simulink model "Arti_DeltaSM_Control_Fricc"  (R2014a)
settings: Solver=ode15s  StartTime=0.0  StopTime=6  FixedStep=0.0005  RelTol=1e-3
PreLoadFcn:
  | Fs=0.001;
  | Fc=0.0005;
undefined symbols (not defined in the file or in its folder): X, Y, Z
libraries: sm_lib x238, Fricciones x15, nesl_utility x10, simulink x3
(part 6 of 6)

== system Arti_DeltaSM_Control_Fricc/DeltaSM/BaseMovil/acopleBaseMovilAntebrazo_3_RIGID/ball_Uniball_1_RIGID ==
  ReferenceFrame : sm_lib/Frames and Transforms/Reference Frame  BlockFunction=simmechanics.library.frames_transforms.reference_frame
  Solid : sm_lib/Body Elements/Solid  InertiaType=Custom  Mass=0.0055458151739754217  MassUnits=kg  CenterOfMass=[-2.6002689251073309e-05 0 0]  CenterOfMassUnits=mm  MomentsOfInertia=[0.091219033457233048 0.091225744336999384 0.12400458181757036]  MomentsOfInertiaUnits=kg*mm^2  ProductsOfInertia=[0 0 0]  ProductsOfInertiaUnits=kg*mm^2  DensityBased=on  Density=1000  DensityUnits=kg/(m^3)  GraphicType=FromGeometry  MarkerShape=Sphere  MarkerSize=10  MarkerSizeUnits=m  GraphicVisPropType=SimpleVisualProperties  GraphicDiffuseColor=[0.89803921568627454 0.89803921568627454 0.89803921568627454]  GraphicSpecularColor=[0.5 0.5 0.5 1.0]  GraphicAmbientColor=[0.15 0.15 0.15 1.0]  GraphicEmissiveColor=[0.0 0.0 0.0 1.0]  GraphicShininess=75  GraphicOpacity=1  GeometryShape=FromFile  RectangleSize=[1 1]  RectangleSizeUnits=m  BrickDimensions=[1 1 1]  BrickDimensionUnits=m  CylinderRadius=1  CylinderRadiusUnits=m  CylinderLength=1  CylinderLengthUnits=m  SphereRadius=1  SphereRadiusUnits=m  EllipsoidRadii=[1 1 1]  EllipsoidRadiiUnits=m  ExtrusionCrossSection=[1 1; -1 1; -1 -1; 1 -1]  ExtrusionCrossSectionUnits=m  ExtrusionLength=1  ExtrusionLengthUnits=m  PolygonNumSides=3  PolygonOuterRadius=1  PolygonOuterRadiusUnits=m  ExtGeomFileType=STL  ExtGeomFileName=ball_Uniball_?? ?????????_sldprt.STL  ExtGeomFileUnits=mm  RevolutionCrossSection=[1 1; 1 -1; 2 -1; 2 1]  RevolutionCrossSectionUnits=m  RevolutionExtent=Full  RevolutionAngle=180  RevolutionAngleUnits=deg  BlockFunction=simmechanics.library.body_elements.solid
  F : PMIOPort  Port=1  Side=Left
  connections:
  ReferenceFrame/RConn1 -- Solid/RConn1 -- F/RConn1

== system Arti_DeltaSM_Control_Fricc/DeltaSM/BaseMovil/acopleBaseMovilAntebrazo_3_RIGID/ball_Uniball_2_RIGID ==
  ReferenceFrame : sm_lib/Frames and Transforms/Reference Frame  BlockFunction=simmechanics.library.frames_transforms.reference_frame
  Solid : sm_lib/Body Elements/Solid  InertiaType=Custom  Mass=0.0055458151739754217  MassUnits=kg  CenterOfMass=[-2.6002689251073309e-05 0 0]  CenterOfMassUnits=mm  MomentsOfInertia=[0.091219033457233048 0.091225744336999384 0.12400458181757036]  MomentsOfInertiaUnits=kg*mm^2  ProductsOfInertia=[0 0 0]  ProductsOfInertiaUnits=kg*mm^2  DensityBased=on  Density=1000  DensityUnits=kg/(m^3)  GraphicType=FromGeometry  MarkerShape=Sphere  MarkerSize=10  MarkerSizeUnits=m  GraphicVisPropType=SimpleVisualProperties  GraphicDiffuseColor=[0.89803921568627454 0.89803921568627454 0.89803921568627454]  GraphicSpecularColor=[0.5 0.5 0.5 1.0]  GraphicAmbientColor=[0.15 0.15 0.15 1.0]  GraphicEmissiveColor=[0.0 0.0 0.0 1.0]  GraphicShininess=75  GraphicOpacity=1  GeometryShape=FromFile  RectangleSize=[1 1]  RectangleSizeUnits=m  BrickDimensions=[1 1 1]  BrickDimensionUnits=m  CylinderRadius=1  CylinderRadiusUnits=m  CylinderLength=1  CylinderLengthUnits=m  SphereRadius=1  SphereRadiusUnits=m  EllipsoidRadii=[1 1 1]  EllipsoidRadiiUnits=m  ExtrusionCrossSection=[1 1; -1 1; -1 -1; 1 -1]  ExtrusionCrossSectionUnits=m  ExtrusionLength=1  ExtrusionLengthUnits=m  PolygonNumSides=3  PolygonOuterRadius=1  PolygonOuterRadiusUnits=m  ExtGeomFileType=STL  ExtGeomFileName=ball_Uniball_?? ?????????_sldprt.STL  ExtGeomFileUnits=mm  RevolutionCrossSection=[1 1; 1 -1; 2 -1; 2 1]  RevolutionCrossSectionUnits=m  RevolutionExtent=Full  RevolutionAngle=180  RevolutionAngleUnits=deg  BlockFunction=simmechanics.library.body_elements.solid
  F : PMIOPort  Port=1  Side=Left
  connections:
  ReferenceFrame/RConn1 -- Solid/RConn1 -- F/RConn1

== matlab function Arti_DeltaSM_Control_Fricc/Cinematica Inversa/Cinematica Inversa ==
  data: Px input; Py input; Pz input; ThetaM1 output; ThetaM2 output; ThetaM3 output; AntThetaM1 input; AntThetaM2 input; AntThetaM3 input
function [ThetaM1, ThetaM2, ThetaM3] = CinInv(Px, Py, Pz,AntThetaM1, AntThetaM2, AntThetaM3)
% function [ThetaM1,ThetaM2,ThetaM3] = CinInv(Px,Py,Pz)
% 
% 
% % 
% % h  = 65.25; % 34.5
% % r  = 34.47;% 65.5;
% % a  = 130; % 130;
% % b  = 275; % 275;
% % 
% % % angulos de las juntas
% % phi = [ 0+pi/2; 2*pi/3+pi/2; 4*pi/3+pi/2];
% % 
% % % respuesta
% % theta = zeros(3,1);
% % 
% % % para cada pata
% % for i=1:3
% %     
% %     % Cinematica inversa para la primera pata
% %     Cxi =  cos(phi(i))*Px + sin(phi(i))*Py + h - r;
% %     Cyi = -sin(phi(i))*Px + cos(phi(i))*Py;
% %     Czi =  Pz;
% %     
% %     t3i = acos( Cyi/b );
% %     K   = ( Cxi^2 + Cyi^2 + Czi^2 - a^2 - b^2 )/( 2*a*b*sin(t3i) );
% %     t2i = acos(K);
% %     
% %     A = a + b*cos(t2i)*sin(t3i);
% %     B = b*sin(t2i)*sin(t3i);
% %     sint1i = (A*Czi - B*Cxi) / ( A*A+B*B );
% %     cost1i = (A*Cxi + B*Czi) / ( A*A+B*B );
% %     
% %     theta(i,1) = atan2( sint1i, cost1i );
% % end
% % 
% % % 
% % ThetaM1=theta(1,1);
% % ThetaM2=theta(2,1);
% % ThetaM3=theta(3,1);
% 
% 
% % % % %%%%%%% %%%%%%%%%%
% % %  %  Parámetros  %
% % 
% r = 34.5; %radio efector final
% R = 65.5;%radio de los ejes de los motores
% l1 = 130; %largo barra 1
% l2 = 275; %largo barra 2
% 
% codo=sign(-1);%codo arriba o cado abajo
% % figure(1)
% %%%%%%%%%%%%%%%%
%  %  Cálculos  %
% % 
% %  for Px=-600+beta:100:600+beta
% %      for Py=-600+beta:100:600+beta
% %          for Pz=-600+beta:100:0+beta
% %  
%  
% PC1 = rotz(0,'deg')*[Px; Py; Pz] + [r-R; 0; 0];
% PC2 = rotz(120,'deg')*[Px; Py; Pz] + [r-R; 0; 0];
% PC3 = rotz(240,'deg')*[Px; Py; Pz] + [r-R; 0; 0];
% 
% %%%%%%%%%%%%%%%%%%%%%%%%%%     THETA 3
% %cosenos de theta 3
% C31=PC1(2)/l2;
% C32=PC2(2)/l2;
% C33=PC3(2)/l2;
% %senos de theta 3
% S31=codo*sqrt(1-C31^2);
% S32=codo*sqrt(1-C32^2);
% S33=codo*sqrt(1-C33^2);
% 
% theta3_1 = atan2(S31,C31);
% theta3_2 = atan2(S32,C32);
% theta3_3 = atan2(S33,C33);
% 
% %%%%%%%%%%%%%%%%%%%%%%%%%      THETA 2
% 
% %cosenos de theta 2
% C21=((PC1(1)^2+PC1(2)^2+PC1(3)^2-l1^2-l2^2)/(2*l1*l2*sin(theta3_1)));
% C22=((PC2(1)^2+PC2(2)^2+PC2(3)^2-l1^2-l2^2)/(2*l1*l2*sin(theta3_2)));
% C23=((PC3(1)^2+PC3(2)^2+PC3(3)^2-l1^2-l2^2)/(2*l1*l2*sin(theta3_3)));
% %senos de theta 2
% S21=codo*sqrt(1-C21^2);
% S22=codo*sqrt(1-C22^2);
% S23=codo*sqrt(1-C23^2);
% 
% theta2_1 = atan2(S21,C21);
% theta2_2 = atan2(S22,C22);
% theta2_3 = atan2(S23,C23);
% 
% CinInv_1 = [l1+l2*sin(theta3_1)*cos(theta2_1), -l2*... 
%     sin(theta3_1)*sin(theta2_1); l2*sin(theta3_1)*sin(theta2_1), ... 
%     l1+l2*sin(theta3_1)*cos(theta2_1)]^-1*[PC1(1), PC1(2)]';
% CinInv_2 = [l1+l2*sin(theta3_2)*cos(theta2_2), -l2*... 
%     sin(theta3_2)*sin(theta2_2); l2*sin(theta3_2)*sin(theta2_2), ... 
%     l1+l2*sin(theta3_2)*cos(theta2_2)]^-1*[PC2(1), PC2(2)]';
% CinInv_3 = [l1+l2*sin(theta3_3)*cos(theta2_3), -l2*... 
%     sin(theta3_3)*sin(theta2_3); l2*sin(theta3_3)*sin(theta2_3), ... 
%     l1+l2*sin(theta3_3)*cos(theta2_3)]^-1*[PC3(1), PC3(2)]';
% 
% 
% cos1_1 = CinInv_1(1,:);
% sin1_1 = CinInv_1(2,:);
% 
% cos1_2 = CinInv_2(1,:);
% sin1_2 = CinInv_2(2,:);
% 
% cos1_3 = CinInv_3(1,:);
% sin1_3 = CinInv_3(2,:);
% 
% ThetaM1 = atan2(sin1_1,cos1_1);
% ThetaM2 = atan2(sin1_2,cos1_2);
% ThetaM3 = atan2(sin1_3,cos1_3);
 
% 
% 
% 
% 
% 
% 
%   if (isreal(theta2_1) && isreal(theta2_2) && isreal(theta2_3))
%  else
%     msgbox('numero imaginario')
%      quit cancel;
%   end
% 
%%%%%%%%%%%%%%%%%%%%%%%%%%%%%%%%%%%%%%%



theta = zeros(3,1);
thetaA = zeros(3,1);
thetaB = zeros(3,1);
alpha = [ 0+pi/2; 2*pi/3+pi/2; 4*pi/3+pi/2];
R  = 65.25; % 34.5
r  = 34.47;% 65.5;
L1  = 130; % 130;
L2  = 275; % 275;

R1=R-r;
Si=1/L1*(-Px^2-Py^2-Pz^2+L2^2-L1^2-R1^2);
for i=1:3
Qi=2*Px*cos(alpha(i))+2*Py*sin(alpha(i));


S1=-2*Pz-sqrt(4*Pz^2+4*R1^2-Si^2+Qi^2*(1-(R1^2)/(L1^2))+Qi*((-2*R1*Si)/L1-4*R1));
C1=-2*R1-Qi*(R1/L1-1)-Si;


theta(i,1) = atan2( S1, C1 )*2;
thetaA(i,1) = atan2( S1, C1 )*2;
thetaB(i,1) = -atan2( S1, -C1 )*2; 

 


 
%   while(theta(i,1)<pi/2)
%  theta(i,1)=theta(i,1)+pi;
%   end
%  while(theta(i,1)>(pi/2))
%  theta(i,1)=theta(i,1)-pi;
%  end

%  if (thetaA(i,1)>pi/2 || thetaB(i,1)>pi/2)
%   theta(i,1)=min(thetaA(i,1),thetaB(i,1)) ;  
%  else
% theta(i,1)=max(thetaA(i,1),thetaB(i,1));
%  end
%  
%  
%  
%  
%  theta(i,1) = (atan2( -S1, C1 )*2)+10*pi;
%   while(theta(i,1)<pi)
%  theta(i,1)=theta(i,1)+pi/2;
%   end
%  while(theta(i,1)>(pi))
%  theta(i,1)=theta(i,1)-pi/2;
%  end

end

if(abs(thetaA(1,1)-AntThetaM1)<abs(thetaB(1,1)-AntThetaM1))
  ThetaM1=thetaA(1,1);  
else
    ThetaM1=thetaB(1,1);  
end


if(abs(thetaA(2,1)-AntThetaM2)<abs(thetaB(2,1)-AntThetaM2))
  ThetaM2=thetaA(2,1);  
else
    ThetaM2=thetaB(2,1);  
end

if(abs(thetaA(3,1)-AntThetaM3)<abs(thetaB(3,1)-AntThetaM3))
  ThetaM3=thetaA(3,1);  
else
    ThetaM3=thetaB(3,1);  
end

% 
% ThetaM1=theta(1,1);
% ThetaM2=theta(2,1);
% ThetaM3=theta(3,1);
